simulink model "main_sim_claw_main_sf"  (Simulink 7.2)
settings: Solver=ode2  SolverMode=SingleTasking  StartTime=0.0  StopTime=tsim_max  FixedStep=dtsim  RelTol=1e-3
StopFcn:
  | %mkplt
undefined symbols (not defined in the file): assertion_time, dtsim, MACH, MACH_gain_mat, MACH_mass_IC, MACH_pos_IC, MACH_pqr_Bmat_IC, MACH_pqr_u_IC, MACH_quat_IC, MACH_throttle_IC, MACH_U_nom_IC, MACH_vel_Bmat_IC, MACH_vel_cvdnom_IC, MACH_vel_IC, MACH_vel_uold_IC, max_LOS_rate, target_pos_IC, target_vel_IC, trac_params, u_llim, u_ulim, use_variable_mass, x_trac_IC
libraries: model_lib x8, mach_lib x5, simulink x3, models x1, utility_lib x1
(part 2 of 2)

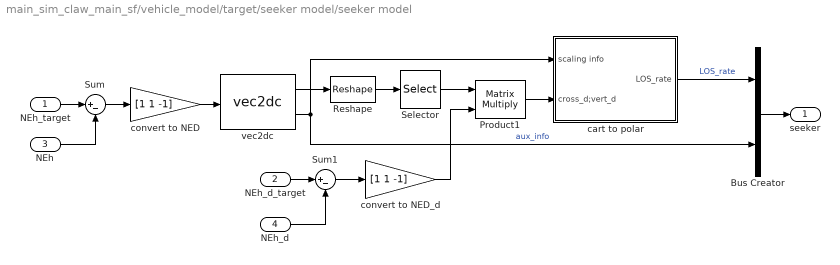
== system main_sim_claw_main_sf/vehicle_model/target/seeker model/seeker model ==
  NEh_target : Inport  OutDataType=sfix(16)  OutScaling=2^0
  NEh_d_target : Inport  Port=2  OutDataType=sfix(16)  OutScaling=2^0
  NEh : Inport  Port=3  OutDataType=sfix(16)  OutScaling=2^0
  NEh_d : Inport  Port=4  OutDataType=sfix(16)  OutScaling=2^0
  Bus Creator : BusCreator  Inputs=2
  Product1 : Product  Multiplication=Matrix(*)  OutDataType=sfix(16)  OutScaling=2^0  RndMeth=Zero
  Reshape : Reshape  OutputDimensionality=Customize  OutputDimensions=[3 3]
  Selector : Selector  NumberOfDimensions=2  InputPortWidth=3  IndexOptions=Index vector (dialog),Select all  Indices=2:3,-1  OutputSizes=1
  Sum : Sum  Inputs=|+-  OutDataType=sfix(16)  OutScaling=2^0
  Sum1 : Sum  Inputs=|+-  OutDataType=sfix(16)  OutScaling=2^0
  cart to polar : Subsystem
  convert to NED : Gain  Gain=[1 1 -1]  ParameterDataType=sfix(16)  ParameterScaling=2^0  OutDataType=sfix(16)  OutScaling=2^0
  convert to NED_d : Gain  Gain=[1 1 -1]  ParameterDataType=sfix(16)  ParameterScaling=2^0  OutDataType=sfix(16)  OutScaling=2^0
  vec2dc : utility_lib/vec2dc  SystemSampleTime=-1
  seeker : Outport  OutDataType=sfix(16)  OutScaling=2^0
  wires:
  cart to polar/1(LOS_rate) -> Bus Creator/1  "LOS_rate"
  NEh_d_target/1 -> Sum1/1
  NEh_target/1 -> Sum/1
  NEh_d/1 -> Sum1/2
  NEh/1 -> Sum/2
  convert to NED_d/1 -> Product1/2
  Product1/1 -> cart to polar/2(cross_d;vert_d)
  Sum1/1 -> convert to NED_d/1
  Selector/1 -> Product1/1
  convert to NED/1 -> vec2dc/1
  Sum/1 -> convert to NED/1
  Reshape/1 -> Selector/1
  vec2dc/1 -> Reshape/1
  vec2dc/2 -> cart to polar/1(scaling info), Bus Creator/2  "aux_info"
  Bus Creator/1 -> seeker/1

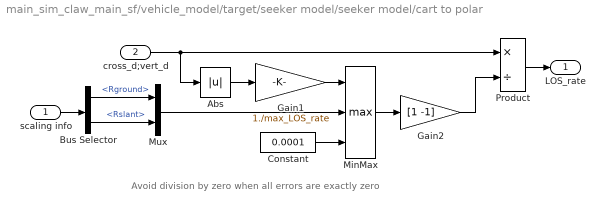
== system main_sim_claw_main_sf/vehicle_model/target/seeker model/seeker model/cart to polar ==
  note: Avoid division by zero when
      | all errors are exactly zero
  scaling info : Inport  OutDataType=sfix(16)  OutScaling=2^0
  cross_d;vert_d : Inport  Port=2  OutDataType=sfix(16)  OutScaling=2^0
  Abs : Abs
  Bus Selector : BusSelector  OutputSignals=Rground,Rslant
  Constant : Constant  Value=0.0001  OutDataType=sfix(16)  OutScaling=2^0
  Gain1 : Gain  Gain=1./max_LOS_rate  ParameterDataType=sfix(16)  ParameterScaling=2^0  OutDataType=sfix(16)  OutScaling=2^0
  Gain2 : Gain  Gain=[1 -1]  ParameterDataType=sfix(16)  ParameterScaling=2^0  OutDataType=sfix(16)  OutScaling=2^0
  MinMax : MinMax  Function=max  Inputs=3  OutDataType=sfix(16)  OutScaling=2^0
  Mux : Mux  Inputs=2
  Product : Product  Inputs=*/  OutDataType=sfix(16)  OutScaling=2^0  RndMeth=Zero
  LOS_rate : Outport  OutDataType=sfix(16)  OutScaling=2^0
  wires:
  Mux/1 -> MinMax/2
  Gain1/1 -> MinMax/1
  Gain2/1 -> Product/2
  MinMax/1 -> Gain2/1
  Abs/1 -> Gain1/1
  Product/1 -> LOS_rate/1
  cross_d;vert_d/1 -> Product/1, Abs/1
  scaling info/1 -> Bus Selector/1
  Bus Selector/1 -> Mux/1  "<Rground>"
  Bus Selector/2 -> Mux/2  "<Rslant>"
  Constant/1 -> MinMax/3
